simulink model "es2_dist"  (R2014a)
settings: Solver=ode45  StartTime=0.0  StopTime=20.0  RelTol=1e-3
values from neighbouring files (symbols this model uses):
  Kr = 2    [es2.m]
libraries: cstblocks x2
settings Model: Creator=HP  LastModifiedBy=HP

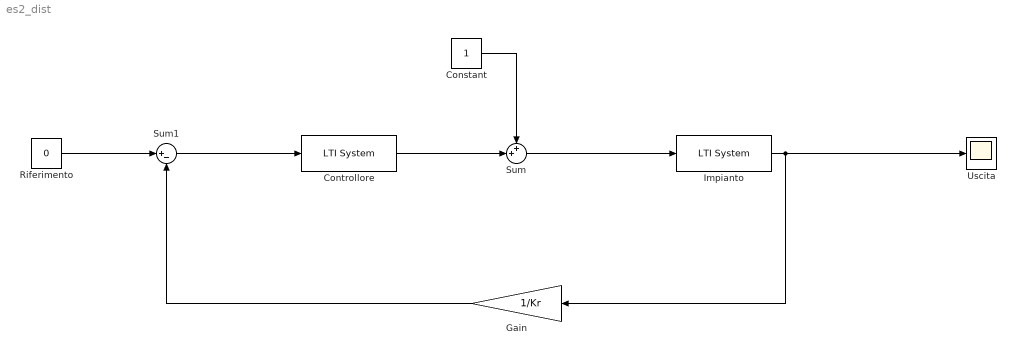
== system es2_dist ==
  Constant : Constant
  Controllore : cstblocks/LTI System  sys=C  IC=[]
  Gain : Gain  Gain=1/Kr
  Impianto : cstblocks/LTI System  sys=F  IC=[]
  Riferimento : Constant  Value=0
  Sum : Sum  Inputs=++|
  Sum1 : Sum  Inputs=|+-
  Uscita : Scope
  wires:
  Controllore/1 -> Sum/2
  Sum/1 -> Impianto/1
  Sum1/1 -> Controllore/1
  Gain/1 -> Sum1/2
  Riferimento/1 -> Sum1/1
  Constant/1 -> Sum/1
  Impianto/1 -> Uscita/1, Gain/1
